simulink model "stateflow_naming11"  (R2015b)
settings: Solver=FixedStepDiscrete  StartTime=0.0  StopTime=10.0  RelTol=1e-3
settings Model: Creator=amyyang  LastModifiedBy=amyyang
settings OptimizationCC: DefaultParameterBehavior=Inlined  OptimizeModelRefInitCode=on  LifeSpan=1
settings RTWCC: SystemTargetFile=ert.tlc  GenCodeOnly=on  TemplateMakefile=ert_default_tmf  Description=Embedded Coder  GenerateReport=on  IncludeHyperlinkInReport=on  LaunchReport=on  GenerateTraceInfo=on  GenerateTraceReport=on  GenerateTraceReportSl=on  GenerateTraceReportSf=on  GenerateTraceReportEml=on
settings CodeAppCC: IgnoreCustomStorageClasses=off
settings ERTTargetCC: GenerateSampleERTMain=on  InlinedParameterPlacement=NonHierarchical  ERTCustomFileTemplate=example_file_process.tlc

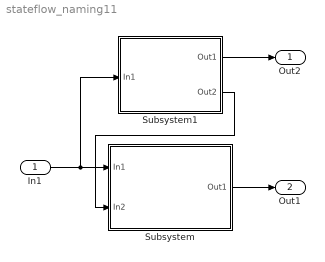
== system stateflow_naming11 ==
  In1 : Inport
  Subsystem : Subsystem  Priority=3
      settings: AttributesFormatString=%<Priority>
  Subsystem1 : Subsystem  Priority=5
      settings: AttributesFormatString=%<Priority>
  Out2 : Outport
  Out1 : Outport  Port=2
  wires:
  Subsystem1/2(Out2) -> Subsystem/2(In2)
  Subsystem/1(Out1) -> Out1/1
  In1/1 -> Subsystem1/1(In1), Subsystem/1(In1)
  Subsystem1/1(Out1) -> Out2/1

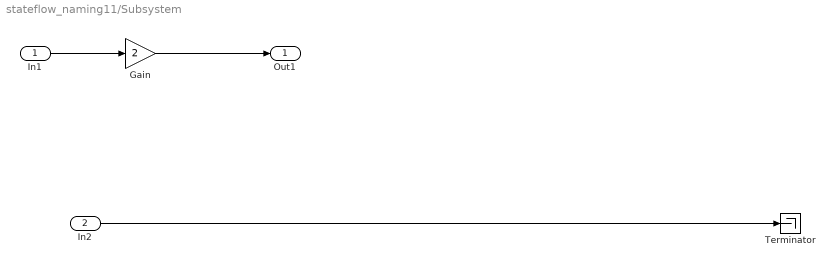
== system stateflow_naming11/Subsystem ==
  In1 : Inport
  In2 : Inport  Port=2
  Gain : Gain  Gain=2
  Terminator : Terminator
  Out1 : Outport
  wires:
  In1/1 -> Gain/1
  In2/1 -> Terminator/1
  Gain/1 -> Out1/1

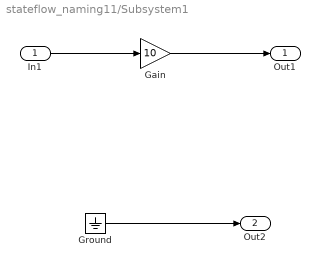
== system stateflow_naming11/Subsystem1 ==
  In1 : Inport
  Gain : Gain  Gain=10
  Ground : Ground
  Out1 : Outport
  Out2 : Outport  Port=2
  wires:
  In1/1 -> Gain/1
  Ground/1 -> Out2/1
  Gain/1 -> Out1/1
